simulink subsystem "Subsystem_Controlador"  (R2023b)
settings: Solver=VariableStepAuto  StartTime=0.0  StopTime=10.0  RelTol=1e-3
settings Model: Creator=Alberto  LastModifiedBy=Alberto

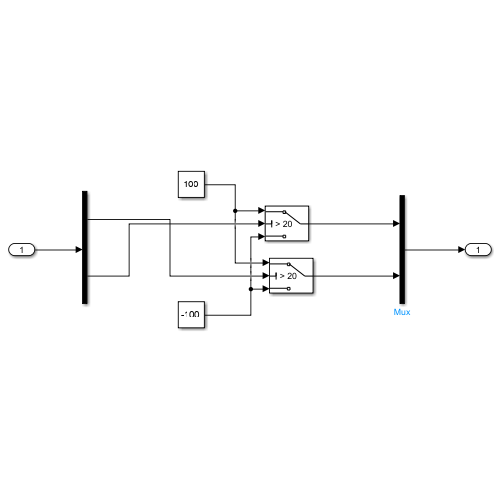
[thumbnail: Simulink's stored preview of the top-level diagram]
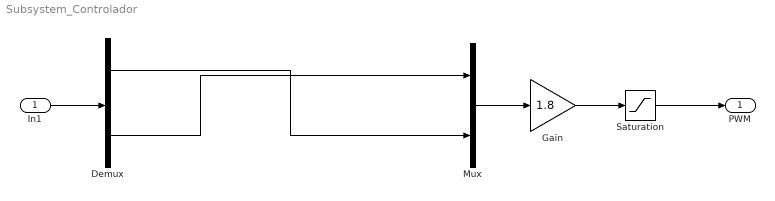
== system Subsystem_Controlador ==
  In1 : Inport
  Demux : Demux  Outputs=2
  Gain : Gain  Gain=1.8
  Mux : Mux  Inputs=2
  Saturation : Saturate  UpperLimit=100  LowerLimit=0
  PWM : Outport
  wires:
  Mux/1 -> Gain/1
  In1/1 -> Demux/1
  Demux/1 -> Mux/2
  Demux/2 -> Mux/1
  Saturation/1 -> PWM/1
  Gain/1 -> Saturation/1
